simulink library "Cl_Lib"  (R2020b)
settings: Solver=VariableStepAuto  StartTime=0.0  StopTime=10.0  RelTol=1e-3
undefined symbols (not defined in the file): N_ClOff, N_ClOn
libraries: $bdroot x1, simulink x1
settings Model: Creator=mtarek-a  LastModifiedBy=mtarek-a

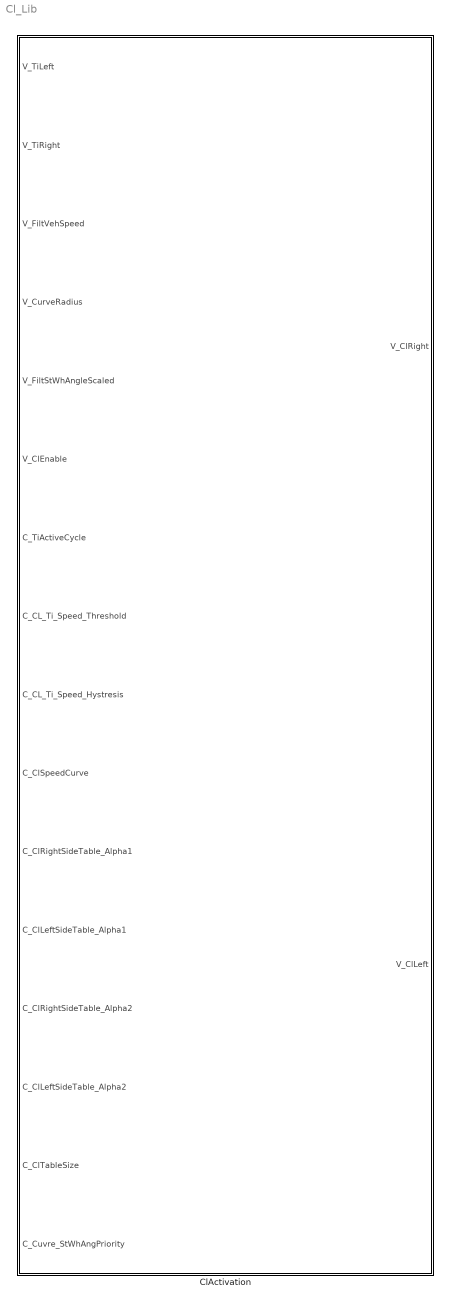
== system Cl_Lib ==
  ClActivation : Subsystem

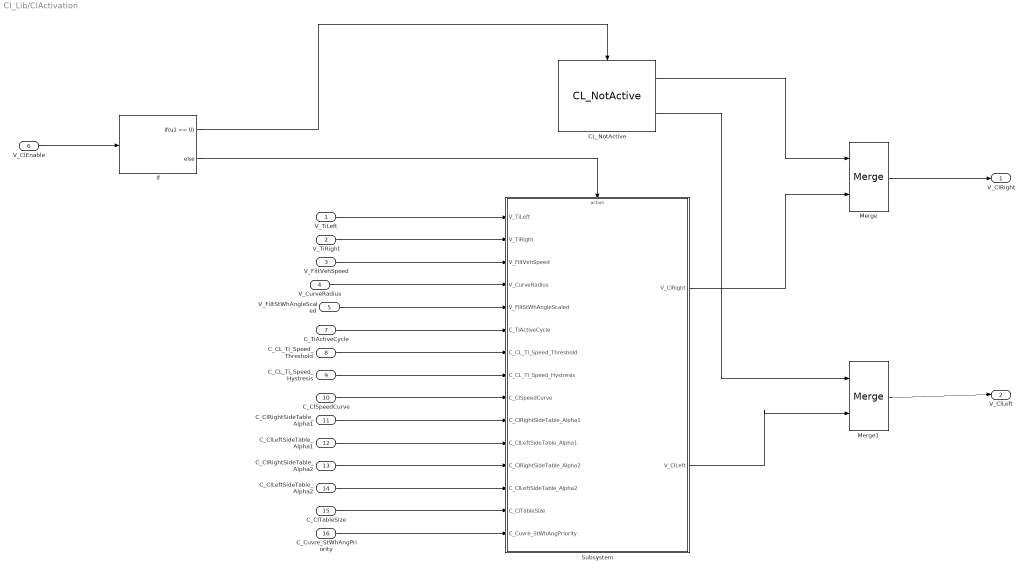
== system Cl_Lib/ClActivation ==
  V_TiLeft : Inport
  V_TiRight : Inport  Port=2
  V_FiltVehSpeed : Inport  Port=3
  V_CurveRadius : Inport  Port=4
  V_FiltStWhAngleScaled : Inport  Port=5
  V_ClEnable : Inport  Port=6
  C_TiActiveCycle : Inport  Port=7
  C_CL_Ti_Speed_Threshold : Inport  Port=8
  C_CL_Ti_Speed_Hystresis : Inport  Port=9
  C_ClSpeedCurve : Inport  Port=10
  C_ClRightSideTable_Alpha1 : Inport  Port=11
  C_ClLeftSideTable_Alpha1 : Inport  Port=12
  C_ClRightSideTable_Alpha2 : Inport  Port=13
  C_ClLeftSideTable_Alpha2 : Inport  Port=14
  C_ClTableSize : Inport  Port=15
  C_Cuvre_StWhAngPriority : Inport  Port=16
  CL_NotActive : $bdroot/ClActivation/Subsystem/FBL_SBL/CL_NotActive  SystemSampleTime=-1  VariantActivationTime=update diagram  Latency=0  AutoFrameSizeCalculation=off
  If : If  IfExpression=u1 == 0
  Merge : Merge
  Merge1 : Merge
  Subsystem : Subsystem
  V_ClRight : Outport
  V_ClLeft : Outport  Port=2
  wires:
  V_TiLeft/1 -> Subsystem/1(V_TiLeft)
  V_TiRight/1 -> Subsystem/2(V_TiRight)
  V_FiltVehSpeed/1 -> Subsystem/3(V_FiltVehSpeed)
  V_CurveRadius/1 -> Subsystem/4(V_CurveRadius)
  V_FiltStWhAngleScaled/1 -> Subsystem/5(V_FiltStWhAngleScaled)
  C_TiActiveCycle/1 -> Subsystem/6(C_TiActiveCycle)
  C_CL_Ti_Speed_Threshold/1 -> Subsystem/7(C_CL_Ti_Speed_Threshold)
  C_CL_Ti_Speed_Hystresis/1 -> Subsystem/8(C_CL_Ti_Speed_Hystresis)
  C_ClSpeedCurve/1 -> Subsystem/9(C_ClSpeedCurve)
  C_ClRightSideTable_Alpha1/1 -> Subsystem/10(C_ClRightSideTable_Alpha1)
  C_ClLeftSideTable_Alpha1/1 -> Subsystem/11(C_ClLeftSideTable_Alpha1)
  C_ClRightSideTable_Alpha2/1 -> Subsystem/12(C_ClRightSideTable_Alpha2)
  C_ClLeftSideTable_Alpha2/1 -> Subsystem/13(C_ClLeftSideTable_Alpha2)
  C_ClTableSize/1 -> Subsystem/14(C_ClTableSize)
  C_Cuvre_StWhAngPriority/1 -> Subsystem/15(C_Cuvre_StWhAngPriority)
  V_ClEnable/1 -> If/1
  CL_NotActive/1 -> Merge/1
  Subsystem/1(V_ClRight) -> Merge/2
  Merge/1 -> V_ClRight/1
  Merge1/1 -> V_ClLeft/1
  CL_NotActive/2 -> Merge1/1
  Subsystem/2(V_ClLeft) -> Merge1/2
  If/1 -> CL_NotActive/Action
  If/2 -> Subsystem/Action

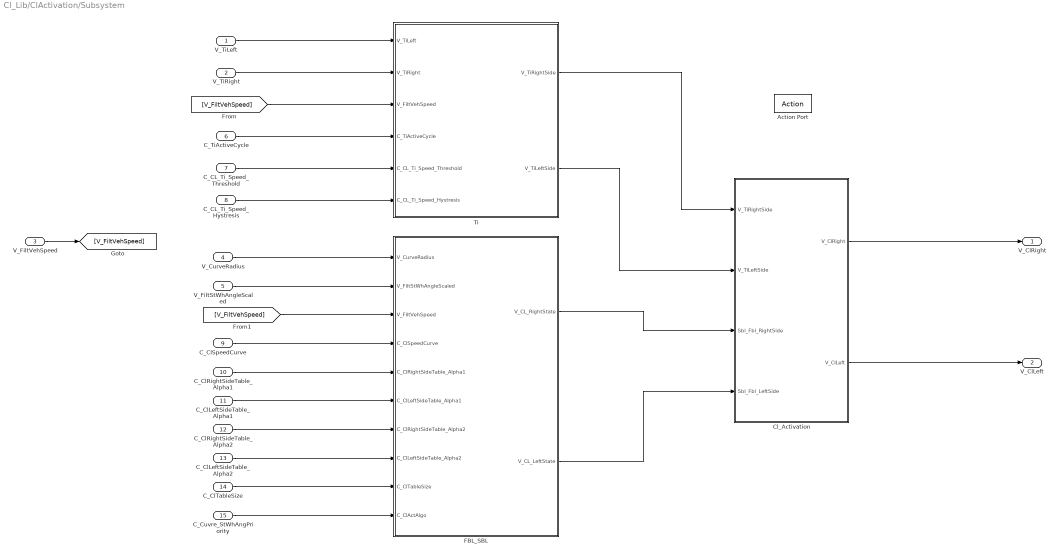
== system Cl_Lib/ClActivation/Subsystem ==
  V_TiLeft : Inport
  V_TiRight : Inport  Port=2
  V_FiltVehSpeed : Inport  Port=3
  V_CurveRadius : Inport  Port=4
  V_FiltStWhAngleScaled : Inport  Port=5
  C_TiActiveCycle : Inport  Port=6
  C_CL_Ti_Speed_Threshold : Inport  Port=7
  C_CL_Ti_Speed_Hystresis : Inport  Port=8
  C_ClSpeedCurve : Inport  Port=9
  C_ClRightSideTable_Alpha1 : Inport  Port=10
  C_ClLeftSideTable_Alpha1 : Inport  Port=11
  C_ClRightSideTable_Alpha2 : Inport  Port=12
  C_ClLeftSideTable_Alpha2 : Inport  Port=13
  C_ClTableSize : Inport  Port=14
  C_Cuvre_StWhAngPriority : Inport  Port=15
  Action Port : ActionPort  ActionPortLabel=else
  Cl_Activation : Subsystem
  FBL_SBL : Subsystem
  Ti : Subsystem
  V_ClRight : Outport
  V_ClLeft : Outport  Port=2
  wires:
  C_CL_Ti_Speed_Threshold/1 -> Ti/5(C_CL_Ti_Speed_Threshold)
  FBL_SBL/2(V_CL_LeftState) -> Cl_Activation/4(Sbl_Fbl_LeftSide)
  C_ClRightSideTable_Alpha2/1 -> FBL_SBL/7(C_ClRightSideTable_Alpha2)
  V_FiltStWhAngleScaled/1 -> FBL_SBL/2(V_FiltStWhAngleScaled)
  C_Cuvre_StWhAngPriority/1 -> FBL_SBL/10(C_ClActAlgo)
  Cl_Activation/2(V_ClLeft) -> V_ClLeft/1
  Ti/1(V_TiRightSide) -> Cl_Activation/1(V_TiRightSide)
  V_FiltVehSpeed/1 -> [V_FiltVehSpeed]
  C_TiActiveCycle/1 -> Ti/4(C_TiActiveCycle)
  C_ClLeftSideTable_Alpha1/1 -> FBL_SBL/6(C_ClLeftSideTable_Alpha1)
  V_TiRight/1 -> Ti/2(V_TiRight)
  FBL_SBL/1(V_CL_RightState) -> Cl_Activation/3(Sbl_Fbl_RightSide)
  [V_FiltVehSpeed] -> Ti/3(V_FiltVehSpeed)
  C_CL_Ti_Speed_Hystresis/1 -> Ti/6(C_CL_Ti_Speed_Hystresis)
  V_CurveRadius/1 -> FBL_SBL/1(V_CurveRadius)
  C_ClRightSideTable_Alpha1/1 -> FBL_SBL/5(C_ClRightSideTable_Alpha1)
  V_TiLeft/1 -> Ti/1(V_TiLeft)
  Ti/2(V_TiLeftSide) -> Cl_Activation/2(V_TiLeftSide)
  C_ClTableSize/1 -> FBL_SBL/9(C_ClTableSize)
  C_ClLeftSideTable_Alpha2/1 -> FBL_SBL/8(C_ClLeftSideTable_Alpha2)
  [V_FiltVehSpeed] -> FBL_SBL/3(V_FiltVehSpeed)
  C_ClSpeedCurve/1 -> FBL_SBL/4(C_ClSpeedCurve)
  Cl_Activation/1(V_ClRight) -> V_ClRight/1

== system Cl_Lib/ClActivation/Subsystem/Cl_Activation ==
  V_TiRightSide : Inport
  V_TiLeftSide : Inport  Port=2
  Sbl_Fbl_RightSide : Inport  Port=3
  Sbl_Fbl_LeftSide : Inport  Port=4
  Logical Operator : Logic  Operator=OR  AllPortsSameDT=off  OutDataTypeStr=boolean
  Logical Operator1 : Logic  Operator=OR  AllPortsSameDT=off  OutDataTypeStr=boolean
  V_ClRight : Outport
  V_ClLeft : Outport  Port=2
  wires:
  Logical Operator/1 -> V_ClRight/1
  Sbl_Fbl_RightSide/1 -> Logical Operator/2
  V_TiRightSide/1 -> Logical Operator/1
  V_TiLeftSide/1 -> Logical Operator1/1
  Sbl_Fbl_LeftSide/1 -> Logical Operator1/2
  Logical Operator1/1 -> V_ClLeft/1

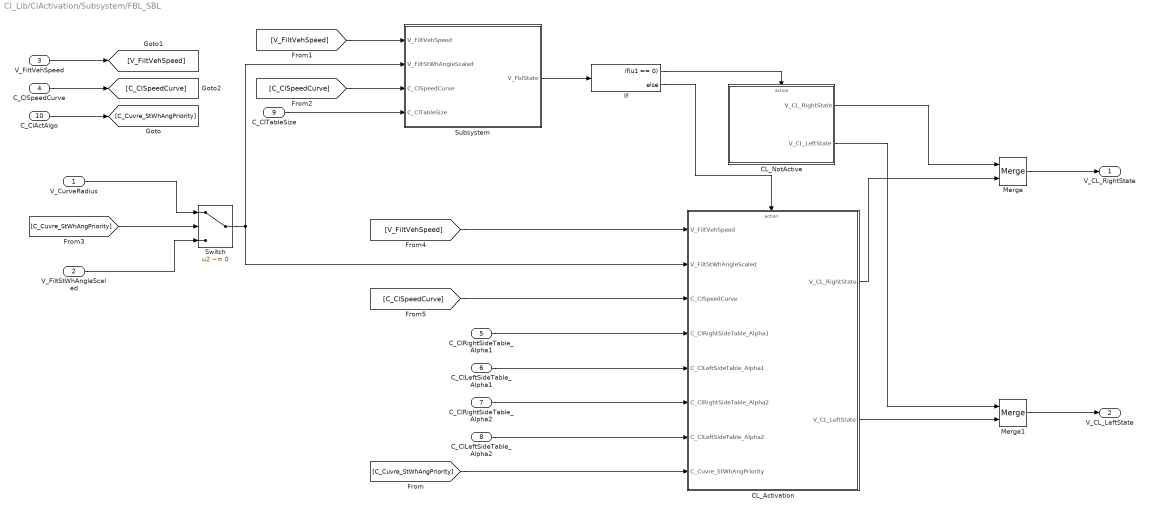
== system Cl_Lib/ClActivation/Subsystem/FBL_SBL ==
  V_CurveRadius : Inport
  V_FiltStWhAngleScaled : Inport  Port=2
  V_FiltVehSpeed : Inport  Port=3
  C_ClSpeedCurve : Inport  Port=4
  C_ClRightSideTable_Alpha1 : Inport  Port=5
  C_ClLeftSideTable_Alpha1 : Inport  Port=6
  C_ClRightSideTable_Alpha2 : Inport  Port=7
  C_ClLeftSideTable_Alpha2 : Inport  Port=8
  C_ClTableSize : Inport  Port=9
  C_ClActAlgo : Inport  Port=10
  CL_Activation : Subsystem
  CL_NotActive : Subsystem
  If : If  IfExpression=u1 == 0
  Merge : Merge
  Merge1 : Merge
  Subsystem : Subsystem
  Switch : Switch  Criteria=u2 ~= 0
  V_CL_RightState : Outport
  V_CL_LeftState : Outport  Port=2
  wires:
  If/2 -> CL_Activation/Action
  C_ClSpeedCurve/1 -> [C_ClSpeedCurve]
  C_ClLeftSideTable_Alpha2/1 -> CL_Activation/7(C_ClLeftSideTable_Alpha2)
  Merge1/1 -> V_CL_LeftState/1
  [C_ClSpeedCurve] -> Subsystem/3(C_ClSpeedCurve)
  Subsystem/1(V_FblState) -> If/1
  If/1 -> CL_NotActive/Action
  [V_FiltVehSpeed] -> Subsystem/1(V_FiltVehSpeed)
  C_ClTableSize/1 -> Subsystem/4(C_ClTableSize)
  C_ClRightSideTable_Alpha1/1 -> CL_Activation/4(C_ClRightSideTable_Alpha1)
  Merge/1 -> V_CL_RightState/1
  CL_Activation/1(V_CL_RightState) -> Merge/2
  CL_Activation/2(V_CL_LeftState) -> Merge1/2
  [C_ClSpeedCurve] -> CL_Activation/3(C_ClSpeedCurve)
  CL_NotActive/2(V_CL_LeftState) -> Merge1/1
  C_ClRightSideTable_Alpha2/1 -> CL_Activation/6(C_ClRightSideTable_Alpha2)
  C_ClLeftSideTable_Alpha1/1 -> CL_Activation/5(C_ClLeftSideTable_Alpha1)
  CL_NotActive/1(V_CL_RightState) -> Merge/1
  V_FiltVehSpeed/1 -> [V_FiltVehSpeed]
  Switch/1 -> Subsystem/2(V_FiltStWhAngleScaled), CL_Activation/2(V_FiltStWhAngleScaled)
  [V_FiltVehSpeed] -> CL_Activation/1(V_FiltVehSpeed)
  V_FiltStWhAngleScaled/1 -> Switch/3
  V_CurveRadius/1 -> Switch/1
  C_ClActAlgo/1 -> [C_Cuvre_StWhAngPriority]
  [C_Cuvre_StWhAngPriority] -> CL_Activation/8(C_Cuvre_StWhAngPriority)
  [C_Cuvre_StWhAngPriority] -> Switch/2

== system Cl_Lib/ClActivation/Subsystem/Ti ==
  V_TiLeft : Inport
  V_TiRight : Inport  Port=2
  V_FiltVehSpeed : Inport  Port=3
  C_TiActiveCycle : Inport  Port=4
  C_CL_Ti_Speed_Threshold : Inport  Port=5
  C_CL_Ti_Speed_Hystresis : Inport  Port=6
  Ti_Activatation : Subsystem
  V_TiRightSide : Outport
  V_TiLeftSide : Outport  Port=2
  wires:
  Ti_Activatation/1(V_TiRightSide) -> V_TiRightSide/1
  Ti_Activatation/2(V_TiLeftSide) -> V_TiLeftSide/1
  V_FiltVehSpeed/1 -> Ti_Activatation/3(V_FiltVehSpeed)
  V_TiRight/1 -> Ti_Activatation/2(V_TiRight)
  V_TiLeft/1 -> Ti_Activatation/1(V_TiLeft)
  C_CL_Ti_Speed_Hystresis/1 -> Ti_Activatation/6(C_CL_Ti_Speed_Hystresis)
  C_CL_Ti_Speed_Threshold/1 -> Ti_Activatation/5(C_CL_Ti_Speed_Threshold)
  C_TiActiveCycle/1 -> Ti_Activatation/4(C_TiActiveCycle)

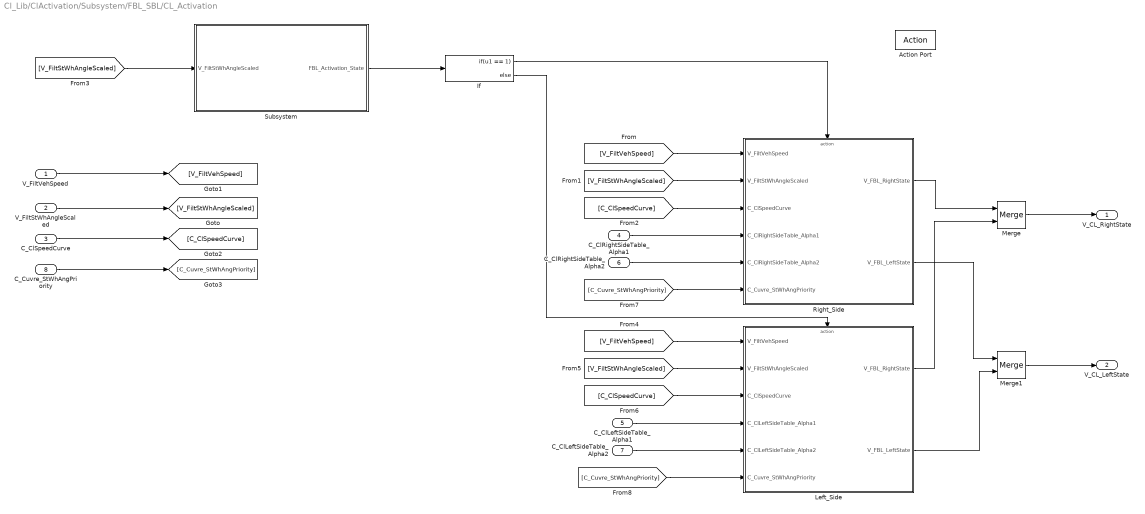
== system Cl_Lib/ClActivation/Subsystem/FBL_SBL/CL_Activation ==
  V_FiltVehSpeed : Inport
  V_FiltStWhAngleScaled : Inport  Port=2
  C_ClSpeedCurve : Inport  Port=3
  C_ClRightSideTable_Alpha1 : Inport  Port=4
  C_ClLeftSideTable_Alpha1 : Inport  Port=5
  C_ClRightSideTable_Alpha2 : Inport  Port=6
  C_ClLeftSideTable_Alpha2 : Inport  Port=7
  C_Cuvre_StWhAngPriority : Inport  Port=8
  Action Port : ActionPort  ActionPortLabel=else
  If : If  IfExpression=u1 == 1
  Left_Side : Subsystem
  Merge : Merge
  Merge1 : Merge
  Right_Side : Subsystem
  Subsystem : Subsystem
  V_CL_RightState : Outport
  V_CL_LeftState : Outport  Port=2
  wires:
  Merge1/1 -> V_CL_LeftState/1
  Merge/1 -> V_CL_RightState/1
  V_FiltVehSpeed/1 -> [V_FiltVehSpeed]
  V_FiltStWhAngleScaled/1 -> [V_FiltStWhAngleScaled]
  C_ClSpeedCurve/1 -> [C_ClSpeedCurve]
  [V_FiltVehSpeed] -> Right_Side/1(V_FiltVehSpeed)
  [V_FiltStWhAngleScaled] -> Right_Side/2(V_FiltStWhAngleScaled)
  [C_ClSpeedCurve] -> Right_Side/3(C_ClSpeedCurve)
  C_ClRightSideTable_Alpha1/1 -> Right_Side/4(C_ClRightSideTable_Alpha1)
  C_ClRightSideTable_Alpha2/1 -> Right_Side/5(C_ClRightSideTable_Alpha2)
  Subsystem/1(FBL_Activation_State) -> If/1
  [V_FiltStWhAngleScaled] -> Subsystem/1(V_FiltStWhAngleScaled)
  If/1 -> Right_Side/Action
  If/2 -> Left_Side/Action
  Right_Side/1(V_FBL_RightState) -> Merge/1
  Left_Side/1(V_FBL_RightState) -> Merge/2
  [V_FiltVehSpeed] -> Left_Side/1(V_FiltVehSpeed)
  [V_FiltStWhAngleScaled] -> Left_Side/2(V_FiltStWhAngleScaled)
  [C_ClSpeedCurve] -> Left_Side/3(C_ClSpeedCurve)
  C_ClLeftSideTable_Alpha1/1 -> Left_Side/4(C_ClLeftSideTable_Alpha1)
  C_ClLeftSideTable_Alpha2/1 -> Left_Side/5(C_ClLeftSideTable_Alpha2)
  Right_Side/2(V_FBL_LeftState) -> Merge1/1
  Left_Side/2(V_FBL_LeftState) -> Merge1/2
  C_Cuvre_StWhAngPriority/1 -> [C_Cuvre_StWhAngPriority]
  [C_Cuvre_StWhAngPriority] -> Right_Side/6(C_Cuvre_StWhAngPriority)
  [C_Cuvre_StWhAngPriority] -> Left_Side/6(C_Cuvre_StWhAngPriority)

== system Cl_Lib/ClActivation/Subsystem/FBL_SBL/CL_NotActive ==
  Action Port : ActionPort  ActionPortLabel=if(u1 == 0)
  Constant : Constant  Value=N_ClOff
  V_CL_RightState : Outport
  V_CL_LeftState : Outport  Port=2
  wires:
  Constant/1 -> V_CL_LeftState/1, V_CL_RightState/1

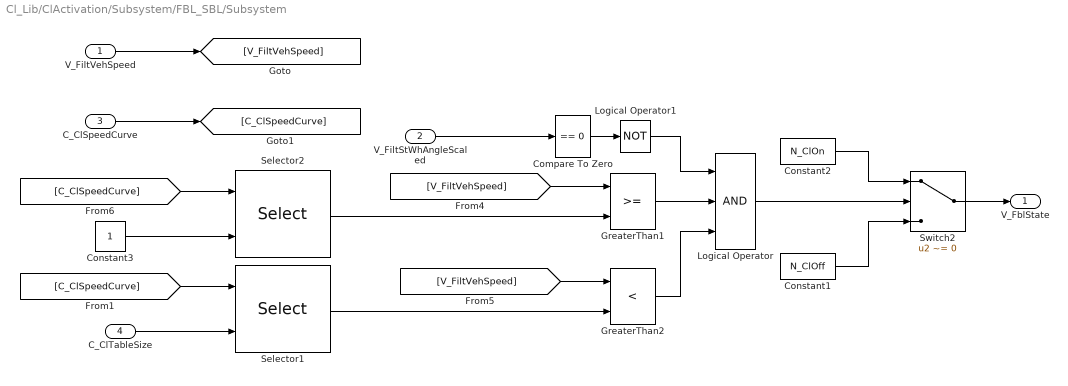
== system Cl_Lib/ClActivation/Subsystem/FBL_SBL/Subsystem ==
  V_FiltVehSpeed : Inport
  V_FiltStWhAngleScaled : Inport  Port=2
  C_ClSpeedCurve : Inport  Port=3
  C_ClTableSize : Inport  Port=4
  Compare To Zero : simulink/Logic and Bit Operations/Compare To Zero  relop===  OutDataTypeStr=boolean
  Constant1 : Constant  Value=N_ClOff
  Constant2 : Constant  Value=N_ClOn
  Constant3 : Constant  OutDataTypeStr=uint8
  GreaterThan1 : RelationalOperator  OutDataTypeStr=boolean  RndMeth=Simplest
  GreaterThan2 : RelationalOperator  Operator=<  OutDataTypeStr=boolean  RndMeth=Simplest
  Logical Operator : Logic  Inputs=3  AllPortsSameDT=off  OutDataTypeStr=boolean
  Logical Operator1 : Logic  Operator=NOT  AllPortsSameDT=off  OutDataTypeStr=boolean
  Selector1 : Selector  IndexOptions=Index vector (port)  Indices=[1 3]  OutputSizes=1
  Selector2 : Selector  IndexOptions=Index vector (port)  Indices=[1 3]  OutputSizes=1
  Switch2 : Switch  Criteria=u2 ~= 0
  V_FblState : Outport
  wires:
  V_FiltStWhAngleScaled/1 -> Compare To Zero/1
  Constant3/1 -> Selector2/2
  Selector2/1 -> GreaterThan1/2
  Logical Operator/1 -> Switch2/2
  Constant1/1 -> Switch2/3
  [V_FiltVehSpeed] -> GreaterThan1/1
  Selector1/1 -> GreaterThan2/2
  [C_ClSpeedCurve] -> Selector1/1
  Constant2/1 -> Switch2/1
  [V_FiltVehSpeed] -> GreaterThan2/1
  [C_ClSpeedCurve] -> Selector2/1
  C_ClTableSize/1 -> Selector1/2
  Switch2/1 -> V_FblState/1
  GreaterThan2/1 -> Logical Operator/3
  GreaterThan1/1 -> Logical Operator/2
  V_FiltVehSpeed/1 -> [V_FiltVehSpeed]
  C_ClSpeedCurve/1 -> [C_ClSpeedCurve]
  Compare To Zero/1 -> Logical Operator1/1
  Logical Operator1/1 -> Logical Operator/1

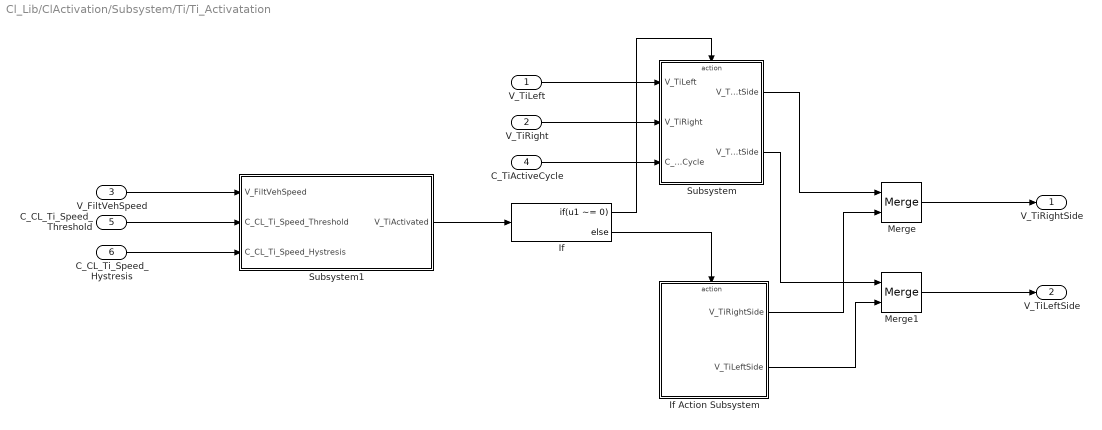
== system Cl_Lib/ClActivation/Subsystem/Ti/Ti_Activatation ==
  V_TiLeft : Inport
  V_TiRight : Inport  Port=2
  V_FiltVehSpeed : Inport  Port=3
  C_TiActiveCycle : Inport  Port=4
  C_CL_Ti_Speed_Threshold : Inport  Port=5
  C_CL_Ti_Speed_Hystresis : Inport  Port=6
  If : If  IfExpression=u1 ~= 0
  If Action Subsystem : Subsystem  TreatAsAtomicUnit=on
  Merge : Merge
  Merge1 : Merge
  Subsystem : Subsystem
  Subsystem1 : Subsystem
  V_TiRightSide : Outport
  V_TiLeftSide : Outport  Port=2
  wires:
  If/1 -> Subsystem/Action
  V_TiRight/1 -> Subsystem/2(V_TiRight)
  Merge/1 -> V_TiRightSide/1
  C_CL_Ti_Speed_Hystresis/1 -> Subsystem1/3(C_CL_Ti_Speed_Hystresis)
  C_TiActiveCycle/1 -> Subsystem/3(C_TiActiveCycle)
  Subsystem1/1(V_TiActivated) -> If/1
  C_CL_Ti_Speed_Threshold/1 -> Subsystem1/2(C_CL_Ti_Speed_Threshold)
  V_TiLeft/1 -> Subsystem/1(V_TiLeft)
  V_FiltVehSpeed/1 -> Subsystem1/1(V_FiltVehSpeed)
  If/2 -> If Action Subsystem/Action
  Merge1/1 -> V_TiLeftSide/1
  Subsystem/1(V_TiRightSide) -> Merge/1
  If Action Subsystem/1(V_TiRightSide) -> Merge/2
  Subsystem/2(V_TiLeftSide) -> Merge1/1
  If Action Subsystem/2(V_TiLeftSide) -> Merge1/2

== system Cl_Lib/ClActivation/Subsystem/FBL_SBL/CL_Activation/Left_Side ==
  V_FiltVehSpeed : Inport
  V_FiltStWhAngleScaled : Inport  Port=2
  C_ClSpeedCurve : Inport  Port=3
  C_ClLeftSideTable_Alpha1 : Inport  Port=4
  C_ClLeftSideTable_Alpha2 : Inport  Port=5
  C_Cuvre_StWhAngPriority : Inport  Port=6
  Action Port : ActionPort
  Calc_StateLeftSide : Subsystem
  Constant1 : Constant  Value=N_ClOff
  Curving_CL_LeftSide : Subsystem
  V_FBL_RightState : Outport
  V_FBL_LeftState : Outport  Port=2
  wires:
  Curving_CL_LeftSide/2(V_Alpha2_LeftSide_State) -> Calc_StateLeftSide/3(V_Alpha2_LeftSide_State)
  Curving_CL_LeftSide/1(V_Alpha1_LeftSide_State) -> Calc_StateLeftSide/2(V_Alpha1_LeftSide_State)
  Calc_StateLeftSide/1(V_FBL_LeftState) -> V_FBL_LeftState/1
  V_FiltVehSpeed/1 -> Curving_CL_LeftSide/1(V_FiltVehSpeed)
  C_ClSpeedCurve/1 -> Curving_CL_LeftSide/2(C_ClSpeedCurve)
  C_ClLeftSideTable_Alpha1/1 -> Curving_CL_LeftSide/3(C_ClLeftSideTable_Alpha1)
  C_ClLeftSideTable_Alpha2/1 -> Curving_CL_LeftSide/4(C_ClLeftSideTable_Alpha2)
  V_FiltStWhAngleScaled/1 -> Calc_StateLeftSide/1(V_FiltStWhAngleScaled)
  Constant1/1 -> V_FBL_RightState/1
  C_Cuvre_StWhAngPriority/1 -> Calc_StateLeftSide/4(C_Cuvre_StWhAngPriority)

== system Cl_Lib/ClActivation/Subsystem/FBL_SBL/CL_Activation/Right_Side ==
  V_FiltVehSpeed : Inport
  V_FiltStWhAngleScaled : Inport  Port=2
  C_ClSpeedCurve : Inport  Port=3
  C_ClRightSideTable_Alpha1 : Inport  Port=4
  C_ClRightSideTable_Alpha2 : Inport  Port=5
  C_Cuvre_StWhAngPriority : Inport  Port=6
  Action Port : ActionPort
  Calc_StateRightSide : Subsystem
  Constant : Constant  Value=N_ClOff
  Curving_CL_RightSide : Subsystem
  V_FBL_RightState : Outport
  V_FBL_LeftState : Outport  Port=2
  wires:
  Calc_StateRightSide/1(V_FBL_RightState) -> V_FBL_RightState/1
  Constant/1 -> V_FBL_LeftState/1
  V_FiltVehSpeed/1 -> Curving_CL_RightSide/1(V_FiltVehSpeed)
  C_ClSpeedCurve/1 -> Curving_CL_RightSide/2(C_ClSpeedCurve)
  C_ClRightSideTable_Alpha1/1 -> Curving_CL_RightSide/3(C_ClRightSideTable_Alpha1)
  C_ClRightSideTable_Alpha2/1 -> Curving_CL_RightSide/4(C_ClRightSideTable_Alpha2)
  Curving_CL_RightSide/1(V_Alpha1_RighSide_State) -> Calc_StateRightSide/2(V_Alpha1_RighSide_State)
  Curving_CL_RightSide/2(V_Alpha2_RighSide_State) -> Calc_StateRightSide/3(V_Alpha2_RighSide_State)
  V_FiltStWhAngleScaled/1 -> Calc_StateRightSide/1(V_FiltStWhAngleScaled)
  C_Cuvre_StWhAngPriority/1 -> Calc_StateRightSide/4(C_Cuvre_StWhAngPriority)

== system Cl_Lib/ClActivation/Subsystem/FBL_SBL/CL_Activation/Subsystem ==
  V_FiltStWhAngleScaled : Inport
  Constant1 : Constant  Value=0  OutDataTypeStr=boolean
  Constant2 : Constant  Value=N_ClOff
  Constant4 : Constant  Value=N_ClOn
  Relational Operator : RelationalOperator  OutDataTypeStr=boolean  RndMeth=Simplest
  Switch : Switch  Criteria=u2 ~= 0
  FBL_Activation_State : Outport
  wires:
  Relational Operator/1 -> Switch/2
  Constant2/1 -> Switch/3
  Switch/1 -> FBL_Activation_State/1
  Constant1/1 -> Relational Operator/2
  V_FiltStWhAngleScaled/1 -> Relational Operator/1
  Constant4/1 -> Switch/1

== system Cl_Lib/ClActivation/Subsystem/Ti/Ti_Activatation/If Action Subsystem ==
  Action Port : ActionPort
  Constant1 : Constant  Value=N_ClOff
  V_TiRightSide : Outport
  V_TiLeftSide : Outport  Port=2
  wires:
  Constant1/1 -> V_TiLeftSide/1, V_TiRightSide/1

== system Cl_Lib/ClActivation/Subsystem/Ti/Ti_Activatation/Subsystem ==
  V_TiLeft : Inport
  V_TiRight : Inport  Port=2
  C_TiActiveCycle : Inport  Port=3
  Action Port : ActionPort
  Ti_LeftSide : Subsystem
  Ti_RightSide : Subsystem
  V_TiRightSide : Outport
  V_TiLeftSide : Outport  Port=2
  wires:
  V_TiLeft/1 -> Ti_LeftSide/1(V_TiLeft)
  V_TiRight/1 -> Ti_RightSide/1(V_TiRight)
  C_TiActiveCycle/1 -> [C_TiActiveCycle]
  [C_TiActiveCycle] -> Ti_RightSide/2(C_TiActiveCycle)
  [C_TiActiveCycle] -> Ti_LeftSide/2(C_TiActiveCycle)
  Ti_RightSide/1(V_TiActive) -> V_TiRightSide/1
  Ti_LeftSide/1(V_TiActive) -> V_TiLeftSide/1

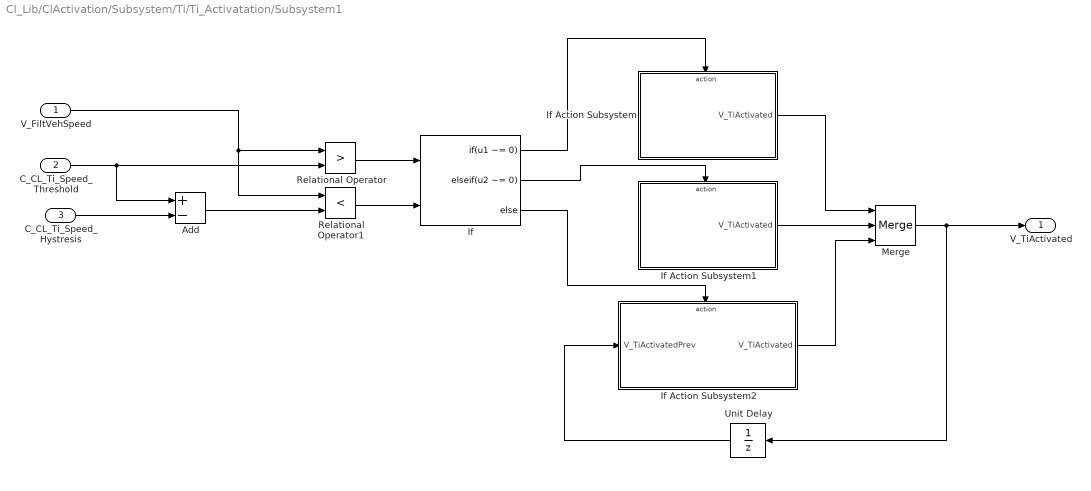
== system Cl_Lib/ClActivation/Subsystem/Ti/Ti_Activatation/Subsystem1 ==
  V_FiltVehSpeed : Inport
  C_CL_Ti_Speed_Threshold : Inport  Port=2
  C_CL_Ti_Speed_Hystresis : Inport  Port=3
  Add : Sum  Inputs=+-
  If : If  NumInputs=2  IfExpression=u1 ~= 0  ElseIfExpressions=u2 ~= 0
  If Action Subsystem : Subsystem  TreatAsAtomicUnit=on
  If Action Subsystem1 : Subsystem  TreatAsAtomicUnit=on
  If Action Subsystem2 : Subsystem  TreatAsAtomicUnit=on
  Merge : Merge  Inputs=3
  Relational Operator : RelationalOperator  Operator=>  OutDataTypeStr=boolean  RndMeth=Simplest
  Relational Operator1 : RelationalOperator  Operator=<  OutDataTypeStr=boolean  RndMeth=Simplest
  Unit Delay : UnitDelay  SampleTime=-1  HasFrameUpgradeWarning=on
  V_TiActivated : Outport
  wires:
  C_CL_Ti_Speed_Hystresis/1 -> Add/2
  V_FiltVehSpeed/1 -> Relational Operator/1, Relational Operator1/1
  C_CL_Ti_Speed_Threshold/1 -> Add/1, Relational Operator/2
  Add/1 -> Relational Operator1/2
  Merge/1 -> V_TiActivated/1, Unit Delay/1
  If Action Subsystem2/1(V_TiActivated) -> Merge/3
  Relational Operator/1 -> If/1
  Relational Operator1/1 -> If/2
  If Action Subsystem1/1(V_TiActivated) -> Merge/2
  If Action Subsystem/1(V_TiActivated) -> Merge/1
  If/2 -> If Action Subsystem1/Action
  If/1 -> If Action Subsystem/Action
  If/3 -> If Action Subsystem2/Action
  Unit Delay/1 -> If Action Subsystem2/1(V_TiActivatedPrev)

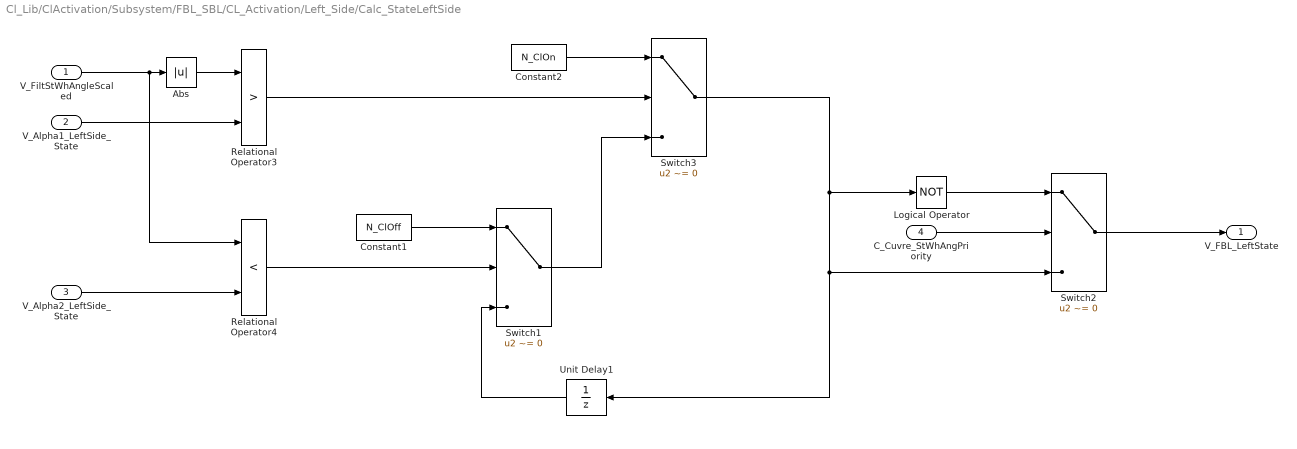
== system Cl_Lib/ClActivation/Subsystem/FBL_SBL/CL_Activation/Left_Side/Calc_StateLeftSide ==
  V_FiltStWhAngleScaled : Inport
  V_Alpha1_LeftSide_State : Inport  Port=2
  V_Alpha2_LeftSide_State : Inport  Port=3
  C_Cuvre_StWhAngPriority : Inport  Port=4
  Abs : Abs
  Constant1 : Constant  Value=N_ClOff
  Constant2 : Constant  Value=N_ClOn
  Logical Operator : Logic  Operator=NOT  AllPortsSameDT=off  OutDataTypeStr=boolean
  Relational Operator3 : RelationalOperator  Operator=>  OutDataTypeStr=boolean  RndMeth=Nearest
  Relational Operator4 : RelationalOperator  Operator=<  OutDataTypeStr=boolean  RndMeth=Nearest
  Switch1 : Switch  Criteria=u2 ~= 0
  Switch2 : Switch  Criteria=u2 ~= 0
  Switch3 : Switch  Criteria=u2 ~= 0
  Unit Delay1 : UnitDelay  SampleTime=-1  HasFrameUpgradeWarning=on
  V_FBL_LeftState : Outport
  wires:
  V_FiltStWhAngleScaled/1 -> Relational Operator4/1, Abs/1
  V_Alpha1_LeftSide_State/1 -> Relational Operator3/2
  Relational Operator3/1 -> Switch3/2
  Constant2/1 -> Switch3/1
  V_Alpha2_LeftSide_State/1 -> Relational Operator4/2
  Relational Operator4/1 -> Switch1/2
  Constant1/1 -> Switch1/1
  Unit Delay1/1 -> Switch1/3
  Switch1/1 -> Switch3/3
  Logical Operator/1 -> Switch2/1
  Switch2/1 -> V_FBL_LeftState/1
  C_Cuvre_StWhAngPriority/1 -> Switch2/2
  Switch3/1 -> Logical Operator/1, Unit Delay1/1, Switch2/3
  Abs/1 -> Relational Operator3/1

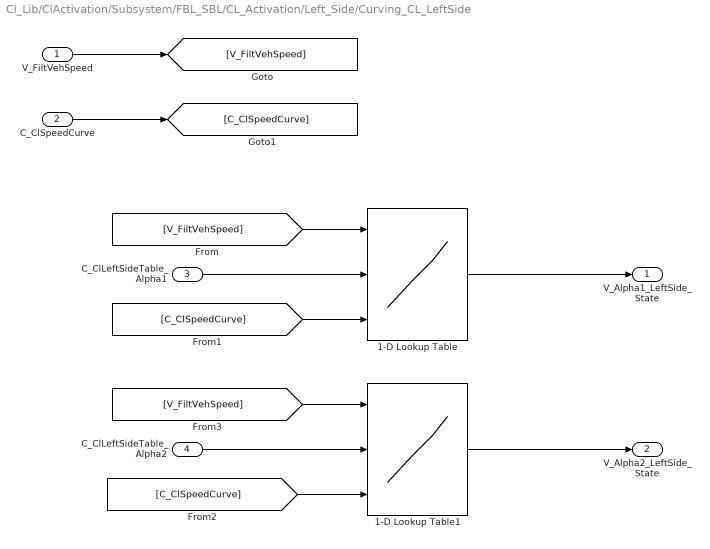
== system Cl_Lib/ClActivation/Subsystem/FBL_SBL/CL_Activation/Left_Side/Curving_CL_LeftSide ==
  V_FiltVehSpeed : Inport
  C_ClSpeedCurve : Inport  Port=2
  C_ClLeftSideTable_Alpha1 : Inport  Port=3
  C_ClLeftSideTable_Alpha2 : Inport  Port=4
  1-D Lookup Table : Lookup_n-D  NumberOfTableDimensions=1  BreakpointsForDimension1Source=Input port  BreakpointsForDimension1=[-5:5]  TableSource=Input port  Table=tanh([-5:5])  ExtrapMethod=Clip  UseLastTableValue=on  InternalRulePriority=Speed  OutDataTypeStr=Inherit: Inherit from 'Table data'  RndMeth=Simplest  InputSameDT=on
      settings: InputPortMap=u0,p221,p5
  1-D Lookup Table1 : Lookup_n-D  NumberOfTableDimensions=1  BreakpointsForDimension1Source=Input port  BreakpointsForDimension1=[-5:5]  TableSource=Input port  Table=tanh([-5:5])  ExtrapMethod=Clip  UseLastTableValue=on  InternalRulePriority=Speed  OutDataTypeStr=Inherit: Inherit from 'Table data'  RndMeth=Simplest  InputSameDT=on
      settings: InputPortMap=u0,p221,p5
  V_Alpha1_LeftSide_State : Outport
  V_Alpha2_LeftSide_State : Outport  Port=2
  wires:
  V_FiltVehSpeed/1 -> [V_FiltVehSpeed]
  [V_FiltVehSpeed] -> 1-D Lookup Table/1
  C_ClSpeedCurve/1 -> [C_ClSpeedCurve]
  [C_ClSpeedCurve] -> 1-D Lookup Table/3
  [C_ClSpeedCurve] -> 1-D Lookup Table1/3
  C_ClLeftSideTable_Alpha1/1 -> 1-D Lookup Table/2
  C_ClLeftSideTable_Alpha2/1 -> 1-D Lookup Table1/2
  [V_FiltVehSpeed] -> 1-D Lookup Table1/1
  1-D Lookup Table/1 -> V_Alpha1_LeftSide_State/1
  1-D Lookup Table1/1 -> V_Alpha2_LeftSide_State/1

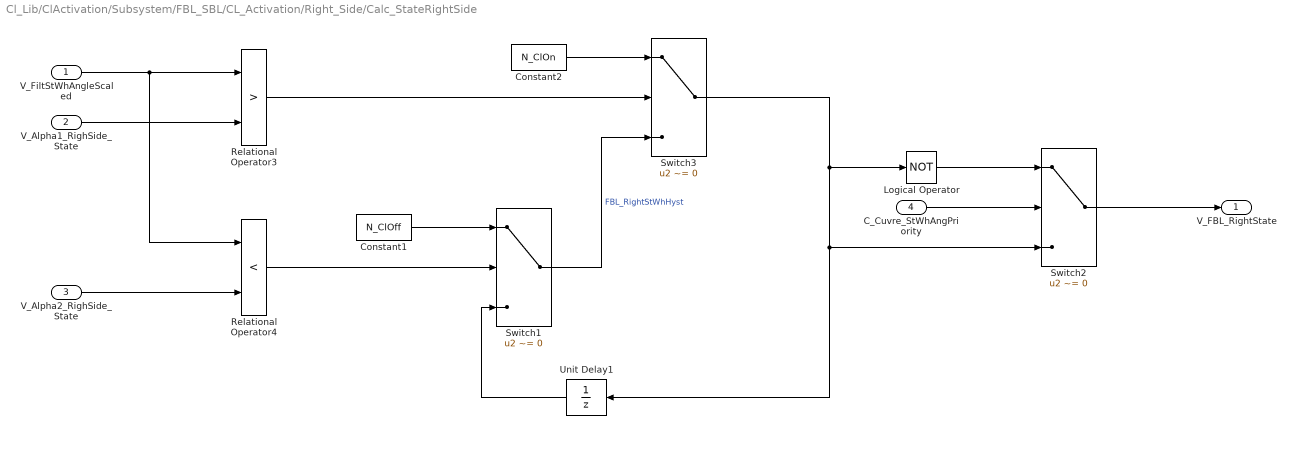
== system Cl_Lib/ClActivation/Subsystem/FBL_SBL/CL_Activation/Right_Side/Calc_StateRightSide ==
  V_FiltStWhAngleScaled : Inport
  V_Alpha1_RighSide_State : Inport  Port=2
  V_Alpha2_RighSide_State : Inport  Port=3
  C_Cuvre_StWhAngPriority : Inport  Port=4
  Constant1 : Constant  Value=N_ClOff
  Constant2 : Constant  Value=N_ClOn
  Logical Operator : Logic  Operator=NOT  AllPortsSameDT=off  OutDataTypeStr=boolean
  Relational Operator3 : RelationalOperator  Operator=>  OutDataTypeStr=boolean  RndMeth=Nearest
  Relational Operator4 : RelationalOperator  Operator=<  OutDataTypeStr=boolean  RndMeth=Nearest
  Switch1 : Switch  Criteria=u2 ~= 0
  Switch2 : Switch  Criteria=u2 ~= 0
  Switch3 : Switch  Criteria=u2 ~= 0
  Unit Delay1 : UnitDelay  SampleTime=-1  HasFrameUpgradeWarning=on
  V_FBL_RightState : Outport
  wires:
  V_Alpha1_RighSide_State/1 -> Relational Operator3/2
  Relational Operator3/1 -> Switch3/2
  Constant2/1 -> Switch3/1
  Switch3/1 -> Logical Operator/1, Switch2/3, Unit Delay1/1
  V_Alpha2_RighSide_State/1 -> Relational Operator4/2
  Relational Operator4/1 -> Switch1/2
  Constant1/1 -> Switch1/1
  Unit Delay1/1 -> Switch1/3
  Switch1/1 -> Switch3/3  "FBL_RightStWhHyst"
  Switch2/1 -> V_FBL_RightState/1
  C_Cuvre_StWhAngPriority/1 -> Switch2/2
  Logical Operator/1 -> Switch2/1
  V_FiltStWhAngleScaled/1 -> Relational Operator3/1, Relational Operator4/1

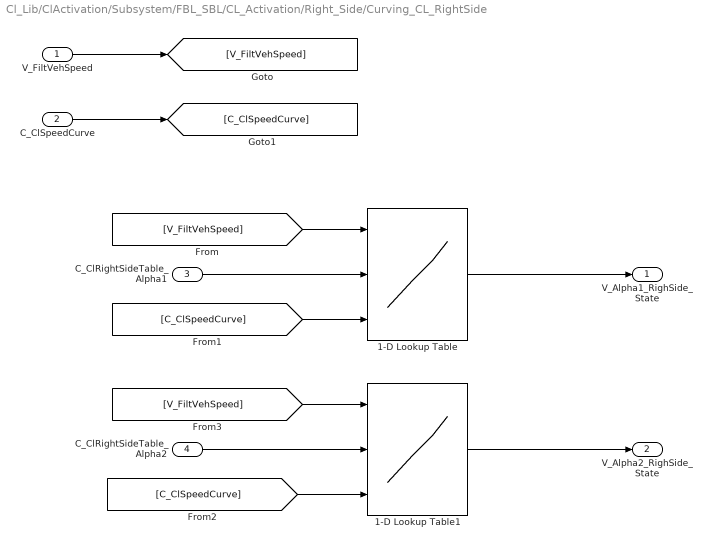
== system Cl_Lib/ClActivation/Subsystem/FBL_SBL/CL_Activation/Right_Side/Curving_CL_RightSide ==
  V_FiltVehSpeed : Inport
  C_ClSpeedCurve : Inport  Port=2
  C_ClRightSideTable_Alpha1 : Inport  Port=3
  C_ClRightSideTable_Alpha2 : Inport  Port=4
  1-D Lookup Table : Lookup_n-D  NumberOfTableDimensions=1  BreakpointsForDimension1Source=Input port  BreakpointsForDimension1=[-5:5]  TableSource=Input port  Table=tanh([-5:5])  ExtrapMethod=Clip  UseLastTableValue=on  InternalRulePriority=Speed  OutDataTypeStr=Inherit: Inherit from 'Table data'  RndMeth=Simplest  InputSameDT=on
      settings: InputPortMap=u0,p221,p5
  1-D Lookup Table1 : Lookup_n-D  NumberOfTableDimensions=1  BreakpointsForDimension1Source=Input port  BreakpointsForDimension1=[-5:5]  TableSource=Input port  Table=tanh([-5:5])  ExtrapMethod=Clip  UseLastTableValue=on  InternalRulePriority=Speed  OutDataTypeStr=Inherit: Inherit from 'Table data'  RndMeth=Simplest  InputSameDT=on
      settings: InputPortMap=u0,p221,p5
  V_Alpha1_RighSide_State : Outport
  V_Alpha2_RighSide_State : Outport  Port=2
  wires:
  V_FiltVehSpeed/1 -> [V_FiltVehSpeed]
  [V_FiltVehSpeed] -> 1-D Lookup Table/1
  C_ClSpeedCurve/1 -> [C_ClSpeedCurve]
  [C_ClSpeedCurve] -> 1-D Lookup Table/3
  [C_ClSpeedCurve] -> 1-D Lookup Table1/3
  C_ClRightSideTable_Alpha1/1 -> 1-D Lookup Table/2
  C_ClRightSideTable_Alpha2/1 -> 1-D Lookup Table1/2
  [V_FiltVehSpeed] -> 1-D Lookup Table1/1
  1-D Lookup Table/1 -> V_Alpha1_RighSide_State/1
  1-D Lookup Table1/1 -> V_Alpha2_RighSide_State/1

== system Cl_Lib/ClActivation/Subsystem/Ti/Ti_Activatation/Subsystem/Ti_LeftSide ==
  V_TiLeft : Inport
  C_TiActiveCycle : Inport  Port=2
  Chart : Stateflow chart  TreatAsAtomicUnit=on
  V_TiActive : Outport
  wires:
  Chart/1(V_TiActive) -> V_TiActive/1
  C_TiActiveCycle/1 -> Chart/1(TiActiveCycle)
  V_TiLeft/1 -> Chart/2(V_TiSignal)

== system Cl_Lib/ClActivation/Subsystem/Ti/Ti_Activatation/Subsystem/Ti_RightSide ==
  V_TiRight : Inport
  C_TiActiveCycle : Inport  Port=2
  Chart : Stateflow chart  TreatAsAtomicUnit=on
  V_TiActive : Outport
  wires:
  Chart/1(V_TiActive) -> V_TiActive/1
  C_TiActiveCycle/1 -> Chart/1(TiActiveCycle)
  V_TiRight/1 -> Chart/2(V_TiSignal)

== system Cl_Lib/ClActivation/Subsystem/Ti/Ti_Activatation/Subsystem1/If Action Subsystem ==
  Action Port : ActionPort
  Constant : Constant  Value=0  OutDataTypeStr=boolean
  V_TiActivated : Outport
  wires:
  Constant/1 -> V_TiActivated/1

== system Cl_Lib/ClActivation/Subsystem/Ti/Ti_Activatation/Subsystem1/If Action Subsystem1 ==
  Action Port : ActionPort
  Constant : Constant  OutDataTypeStr=boolean
  V_TiActivated : Outport
  wires:
  Constant/1 -> V_TiActivated/1

== system Cl_Lib/ClActivation/Subsystem/Ti/Ti_Activatation/Subsystem1/If Action Subsystem2 ==
  V_TiActivatedPrev : Inport
  Action Port : ActionPort
  V_TiActivated : Outport
  wires:
  V_TiActivatedPrev/1 -> V_TiActivated/1

== stateflow chart Cl_Lib/ClActivation/Subsystem/Ti/Ti_Activatation/Subsystem/Ti_LeftSide/Chart ==
  state TiActiveCycle
    state Off1
      entry:
      V_TiActive=0;
    state Waiting
    state ON
      entry:
      V_TiActive=1;
    (default) -> Off1
    Waiting -> Off1 [order 2] : [after(TiActiveCycle,tick)]
    ON -> Waiting : [(V_TiSignal == 0) ]
    Waiting -> ON [order 1] : [(V_TiSignal == 1) ]
    Off1 -> ON : [(V_TiSignal == 1) ]
  data: TiActiveCycle input; V_TiActive output boolean; V_TiSignal input

== stateflow chart Cl_Lib/ClActivation/Subsystem/Ti/Ti_Activatation/Subsystem/Ti_RightSide/Chart ==
  state TiActiveCycle
    state Off1
      entry:
      V_TiActive=0;
    state Waiting
    state ON
      entry:
      V_TiActive=1;
    (default) -> Off1
    Waiting -> Off1 [order 2] : [after(TiActiveCycle,tick)]
    ON -> Waiting : [(V_TiSignal == 0) ]
    Waiting -> ON [order 1] : [(V_TiSignal == 1) ]
    Off1 -> ON : [(V_TiSignal == 1) ]
  data: TiActiveCycle input; V_TiActive output boolean; V_TiSignal input
